simulink model "pendulum_sim"  (Simulink 7.4)
settings: Solver=ode45  StartTime=0.0  StopTime=Tstop  RelTol=1e-3
values from neighbouring files (symbols this model uses):
  beta = 0.2    [grabtheball.m]    (also in pendulum_init.m = 0.5)
  C = hybcon(S,Q,N,limits,refs)    [binary_inputs_sim.m]    (also in bm99benchmark.m; bm99norm2.m; bm99sim.m; exp2mld_mimo.m = lincon(model,'track',cost,interval,limits))
  g = 9.8    [bball.m]    (also in pendulum_init.m = 9.81)
  len = 0.5    [pendulum_init.m]
  mass = 1    [pendulum_init.m]
  x0 = [5 0]'    [bball.m]    (also in binary_inputs_sim.m = [0;0]; bm99sim.m = [0;0]; exp2mld_mimo.m = zeros(nx,1); grabtheball.m = [0 0 5 5 0 0]')
libraries: hyblib x1
settings Model: Creator=bemporad  LastModifiedBy=bemporad
settings DataIOCC: SignalLoggingName=sigsOut
settings DebuggingCC: SaveWithParameterizedLinksMsg=none  SignalResolutionControl=TryResolveAllWithWarning  SolverPrmCheckMsg=none  MultiTaskDSMMsg=warning  MultiTaskCondExecSysMsg=none  StrictBusMsg=None
settings HardwareCC: TargetUnknown=on
settings RTWCC: IncludeERTFirstTime=on

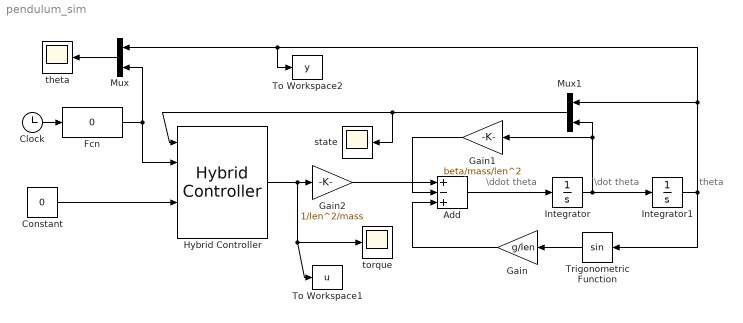
== system pendulum_sim ==
  note: \ddot theta
  note: \dot theta
  note: theta
  Add : Sum  Inputs=+-+
  Clock : Clock
      settings: Decimation=10
  Constant : Constant  Value=0
  Fcn : Fcn  Expr=0
  Gain : Gain  Gain=g/len
  Gain1 : Gain  Gain=beta/mass/len^2
  Gain2 : Gain  Gain=1/len^2/mass
  Hybrid Controller : hyblib/Hybrid Controller  SystemSampleTime=-1  C=C  S=S  tilim=Inf
  Integrator : Integrator  InitialCondition=x0(2)
  Integrator1 : Integrator  InitialCondition=x0(1)
  Mux : Mux  Inputs=2
  Mux1 : Mux  Inputs=2
  To Workspace1 : ToWorkspace  VariableName=u  SampleTime=-1  SaveFormat=Structure With Time
  To Workspace2 : ToWorkspace  VariableName=y  SampleTime=-1  SaveFormat=Structure With Time
  Trigonometric Function : Trigonometry
  state : Scope
      settings: SaveName=ScopeData3
  theta : Scope
      settings: TimeRange=4  YMin=-1  YMax=4  SaveName=ScopeData4
  torque : Scope
      settings: TimeRange=4  YMin=-15  YMax=10  SaveName=ScopeData2
  wires:
  Hybrid Controller/1 -> Gain2/1, torque/1, To Workspace1/1
  Constant/1 -> Hybrid Controller/4
  Mux/1 -> theta/1
  Integrator/1 -> Integrator1/1, Gain1/1, Mux1/2
  Integrator1/1 -> Trigonometric Function/1, Mux1/1, Mux/1, To Workspace2/1
  Trigonometric Function/1 -> Gain/1
  Gain/1 -> Add/3
  Gain1/1 -> Add/2
  Add/1 -> Integrator/1
  Gain2/1 -> Add/1
  Mux1/1 -> state/1, Hybrid Controller/1
  Fcn/1 -> Hybrid Controller/2, Mux/2
  Clock/1 -> Fcn/1
